simulink model "operationalSpaceInverseDynamicsControl_admittance_compact"  (R2021a)
settings: Solver=VariableStepAuto  StartTime=0.0  StopTime=25  RelTol=1e-3
values from neighbouring files (symbols this model uses):
  K = diag([0 10 0 0 0 10])    [assignment13_main.m]
  Kd = 20*diag([10, 10, 10, 10, 10, 10])    [assignment13_main.m]
  Kd_t = 1*diag([10, 10, 10, 10, 10, 10])    [assignment13_main.m]
  Kp = 50*diag([10, 10, 10, 10, 10, 10])    [assignment13_main.m]
  Kp_t = 5*diag([10, 10, 10, 10, 10, 10])    [assignment13_main.m]
  M_d = 0.1*diag([10 10 10 10 10 10])    [assignment13_main.m]
  M_t = 0.05*diag([10 10 10 10 10 10])    [assignment13_main.m]
  x_d_const = [numeric_dk(1:3,4) ... (first row only)    [assignment13_main.m]
libraries: vrlib x1, robotcorelib x1
settings Model: Creator=fabio  LastModifiedBy=fabio

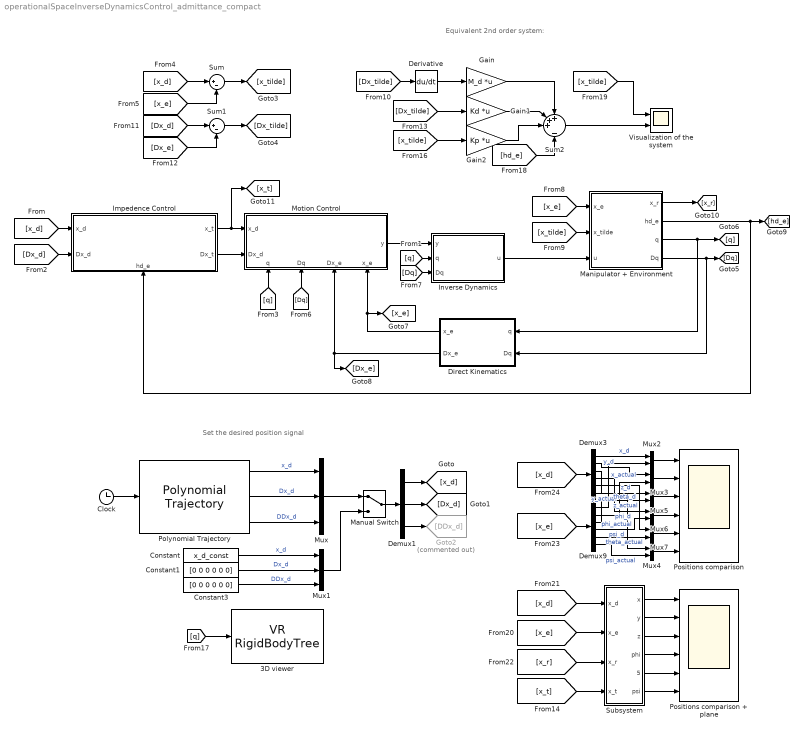
== system operationalSpaceInverseDynamicsControl_admittance_compact ==
  note: Set the desired position signal
  note: Equivalent 2nd order system:
  3D viewer : vrlib/VR RigidBodyTree  RBT=robot  useRBT=off  Ts=0.5  ForceViewerOpen=on
      settings: SourceProductBaseCode=SL
  Clock : Clock
  Constant : Constant  Value=x_d_const
  Constant1 : Constant  Value=[0 0 0 0 0 0]
  Constant3 : Constant  Value=[0 0 0 0 0 0]
  Demux1 : Demux  Outputs=3
  Demux3 : Demux  Outputs=6
  Demux9 : Demux  Outputs=6
  Derivative : Derivative
  Direct Kinematics : Subsystem
  Gain : Gain  Gain=M_d  Multiplication=Matrix(K*u)
  Gain1 : Gain  Gain=Kd  Multiplication=Matrix(K*u)
  Gain2 : Gain  Gain=Kp  Multiplication=Matrix(K*u)
  Goto2 : Goto  Commented=on  GotoTag=DDx_d
  Impedence Control : Subsystem
      settings: PortSchema="{\"entries\":[{\"content\":{\"sides\":[{\"content\":{\"connectorIds\":[\"In1\",\"In2\"]},\"type\":\"ConnectorPlacement.EquallySpacedRectSide\",\"uuid\":\"4a21bbab-43a7-495a-80bb-06e5f1d5644f\"},{\"content\":{\"connectorIds\":[\"Out1\",\"Out2\"],\"side\":\"RIGHT\"},\"type\":\"ConnectorPlacement.EquallySpacedRectSide\",\"uuid\":\"408d256b-dc21-48d5-8048-0ab1741a41e2\"},{\"content\":{\"connectorIds\":[],\"side\":\"TOP\"},\"type\":\"ConnectorPlacement.EquallySpacedRectSide\",\"uuid\":\"05326777-d73e-456a-8a24-eec595721ebb\"},{\"content\":{\"connectorIds\":[\"In3\"],\"side\":\"BOTTOM\"},\"type\":\"ConnectorPlacement.EquallySpacedRectSide\",\"uuid\":\"d6ac4636-ecb5-40e1-909e-b7ba41c5dbf6\"}]},\"type\":\"ConnectorPlacement.EquallySpacedConnector\",\"uuid\":\"f5a6fa07-c06e-4cca-970a-a576f537631e\"}],\"packageUris\":[\"http://schema.mathworks.com/mf0/Connector/R2020b\"],\"version\":\"1.0\"}"
  Inverse Dynamics : Subsystem
  Manipulator + Environment : Subsystem
  Manual Switch : ManualSwitch
  Motion Control : Subsystem
      settings: PortSchema="{\"entries\":[{\"content\":{\"sides\":[{\"content\":{\"connectorIds\":[\"In1\",\"In2\"]},\"type\":\"ConnectorPlacement.EquallySpacedRectSide\",\"uuid\":\"4a21bbab-43a7-495a-80bb-06e5f1d5644f\"},{\"content\":{\"connectorIds\":[\"Out1\"],\"side\":\"RIGHT\"},\"type\":\"ConnectorPlacement.EquallySpacedRectSide\",\"uuid\":\"408d256b-dc21-48d5-8048-0ab1741a41e2\"},{\"content\":{\"connectorIds\":[],\"side\":\"TOP\"},\"type\":\"ConnectorPlacement.EquallySpacedRectSide\",\"uuid\":\"05326777-d73e-456a-8a24-eec595721ebb\"},{\"content\":{\"connectorIds\":[\"In3\",\"In4\",\"In5\",\"In6\"],\"side\":\"BOTTOM\"},\"type\":\"ConnectorPlacement.EquallySpacedRectSide\",\"uuid\":\"d6ac4636-ecb5-40e1-909e-b7ba41c5dbf6\"}]},\"type\":\"ConnectorPlacement.EquallySpacedConnector\",\"uuid\":\"f5a6fa07-c06e-4cca-970a-a576f537631e\"}],\"packageUris\":[\"http://schema.mathworks.com/mf0/Connector/R2020b\"],\"version\":\"1.0\"}"
  Mux : Mux  Inputs=3
  Mux1 : Mux  Inputs=3
  Mux{2..7} (6 alike) : Mux  Inputs=2
  Polynomial Trajectory : robotcorelib/Polynomial Trajectory  WaypointSource=Internal  Waypoints=x_d  TimePoints=[ 0, 10, 20]  TimeInterval=[ 1, 4 ]  Method=Cubic Polynomial  ParameterSource=Internal  VelocityBoundaryCondition=zeros( 6, 3)  AccelerationBoundaryCondition=zeros( 2, 5 )  SimulateUsing=Interpreted execution
  Positions comparison : Scope  NumInputPorts=6
  Positions comparison + plane : Scope  NumInputPorts=6
  Subsystem : Subsystem
  Sum : Sum  Inputs=|+-
  Sum1 : Sum  Inputs=|+-
  Sum2 : Sum  Inputs=+++|-
  Visualization of the system : Scope  NumInputPorts=2
  wires:
  Clock/1 -> Polynomial Trajectory/1
  Polynomial Trajectory/2 -> Mux/2  "Dx_d"
  Polynomial Trajectory/1 -> Mux/1  "x_d"
  Polynomial Trajectory/3 -> Mux/3  "DDx_d"
  Mux/1 -> Manual Switch/1
  Manual Switch/1 -> Demux1/1
  Demux1/1 -> [x_d]
  Demux1/2 -> [Dx_d]
  Demux1/3 -> Goto2/1
  Constant/1 -> Mux1/1  "x_d"
  Constant1/1 -> Mux1/2  "Dx_d"
  Mux1/1 -> Manual Switch/2
  Constant3/1 -> Mux1/3  "DDx_d"
  [q] -> 3D viewer/1
  Manipulator + Environment/4(Dq) -> Direct Kinematics/2(Dq), [Dq]
  Manipulator + Environment/3(q) -> Direct Kinematics/1(q), [q]
  Inverse Dynamics/1(u) -> Manipulator + Environment/3(u)
  [q] -> Inverse Dynamics/2(q)
  [Dq] -> Inverse Dynamics/3(Dq)
  Manipulator + Environment/2(hd_e) -> Impedence Control/3(hd_e), [hd_e]
  Direct Kinematics/2(Dx_e) -> [Dx_e], Motion Control/5(Dx_e)
  Direct Kinematics/1(x_e) -> [x_e], Motion Control/6(x_e)
  [x_d] -> Sum/1
  [x_e] -> Sum/2
  Sum/1 -> [x_tilde]
  [x_e] -> Manipulator + Environment/1(x_e)
  [x_tilde] -> Manipulator + Environment/2(x_tilde)
  [Dx_tilde] -> Derivative/1
  Sum1/1 -> [Dx_tilde]
  [Dx_d] -> Sum1/1
  [Dx_e] -> Sum1/2
  Derivative/1 -> Gain/1
  Gain/1 -> Sum2/1
  [Dx_tilde] -> Gain1/1
  Gain1/1 -> Sum2/2
  [x_tilde] -> Gain2/1
  Gain2/1 -> Sum2/3
  [hd_e] -> Sum2/4
  [x_tilde] -> Visualization of the system/1
  Sum2/1 -> Visualization of the system/2
  [x_d] -> Impedence Control/1(x_d)
  [Dx_d] -> Impedence Control/2(Dx_d)
  Impedence Control/1(x_t) -> [x_t], Motion Control/1(x_d)
  Impedence Control/2(Dx_t) -> Motion Control/2(Dx_d)
  [q] -> Motion Control/3("q  ")
  [Dq] -> Motion Control/4(Dq)
  Motion Control/1(y) -> Inverse Dynamics/1(y)
  Subsystem/5(theta) -> Positions comparison + plane/5
  Subsystem/4(phi) -> Positions comparison + plane/4
  [x_e] -> Subsystem/2(x_e)
  Subsystem/2(y) -> Positions comparison + plane/2
  [x_r] -> Subsystem/3(x_r)
  Subsystem/1(x) -> Positions comparison + plane/1
  Subsystem/3(z) -> Positions comparison + plane/3
  Subsystem/6(psi) -> Positions comparison + plane/6
  [x_d] -> Subsystem/1(x_d)
  [x_e] -> Demux9/1
  Demux9/3 -> Mux5/2  "z_actual"
  Demux9/1 -> Mux2/2  "x_actual"
  [x_d] -> Demux3/1
  Demux3/2 -> Mux3/1  "y_d"
  Demux9/4 -> Mux6/2  "phi_actual"
  Mux7/1 -> Positions comparison/5
  Mux4/1 -> Positions comparison/6
  Demux9/5 -> Mux7/2  "theta_actual"
  Mux2/1 -> Positions comparison/1
  Demux9/6 -> Mux4/2  "psi_actual"
  Demux3/4 -> Mux6/1  "phi_d"
  Mux5/1 -> Positions comparison/3
  Mux6/1 -> Positions comparison/4
  Demux9/2 -> Mux3/2  "y_actual"
  Demux3/6 -> Mux4/1  "psi_d"
  Demux3/1 -> Mux2/1  "x_d"
  Demux3/3 -> Mux5/1  "z_d"
  Mux3/1 -> Positions comparison/2
  Demux3/5 -> Mux7/1  "theta_d"
  Manipulator + Environment/1(x_r) -> [x_r]
  [x_t] -> Subsystem/4(x_t)

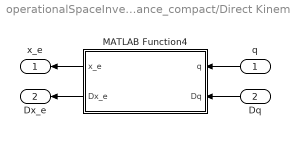
== system operationalSpaceInverseDynamicsControl_admittance_compact/Direct Kinematics ==
  q : Inport
  Dq : Inport  Port=2
  MATLAB Function4 : MATLAB Function  TreatAsAtomicUnit=on
  x_e : Outport
  Dx_e : Outport  Port=2
  wires:
  MATLAB Function4/1(x_e) -> x_e/1
  q/1 -> MATLAB Function4/1(q)
  Dq/1 -> MATLAB Function4/2(Dq)
  MATLAB Function4/2(Dx_e) -> Dx_e/1

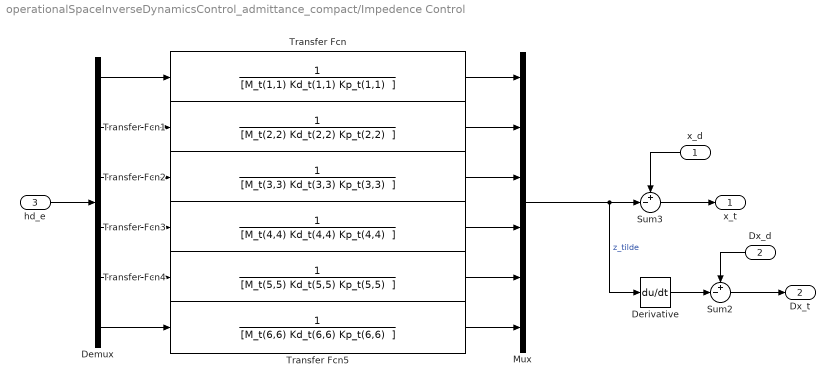
== system operationalSpaceInverseDynamicsControl_admittance_compact/Impedence Control ==
  x_d : Inport
  Dx_d : Inport  Port=2
  hd_e : Inport  Port=3
  Demux : Demux  Outputs=6
  Derivative : Derivative
  Mux : Mux  Inputs=6
  Sum2 : Sum  Inputs=+-|
  Sum3 : Sum  Inputs=+-|
  Transfer Fcn : TransferFcn  Numerator=1  Denominator="[M_t(1,1) Kd_t(1,1) Kp_t(1,1)  ]"
  Transfer Fcn1 : TransferFcn  Numerator=1  Denominator="[M_t(2,2) Kd_t(2,2) Kp_t(2,2)  ]"
  Transfer Fcn2 : TransferFcn  Numerator=1  Denominator="[M_t(3,3) Kd_t(3,3) Kp_t(3,3)  ]"
  Transfer Fcn3 : TransferFcn  Numerator=1  Denominator="[M_t(4,4) Kd_t(4,4) Kp_t(4,4)  ]"
  Transfer Fcn4 : TransferFcn  Numerator=1  Denominator="[M_t(5,5) Kd_t(5,5) Kp_t(5,5)  ]"
  Transfer Fcn5 : TransferFcn  Numerator=1  Denominator="[M_t(6,6) Kd_t(6,6) Kp_t(6,6)  ]"
  x_t : Outport
  Dx_t : Outport  Port=2
  wires:
  x_d/1 -> Sum3/1
  hd_e/1 -> Demux/1
  Demux/1 -> Transfer Fcn/1
  Demux/2 -> Transfer Fcn1/1
  Demux/3 -> Transfer Fcn2/1
  Demux/4 -> Transfer Fcn3/1
  Demux/5 -> Transfer Fcn4/1
  Demux/6 -> Transfer Fcn5/1
  Transfer Fcn/1 -> Mux/1
  Transfer Fcn1/1 -> Mux/2
  Transfer Fcn2/1 -> Mux/3
  Transfer Fcn3/1 -> Mux/4
  Transfer Fcn4/1 -> Mux/5
  Transfer Fcn5/1 -> Mux/6
  Mux/1 -> Derivative/1, Sum3/2  "z_tilde"
  Sum3/1 -> x_t/1
  Sum2/1 -> Dx_t/1
  Dx_d/1 -> Sum2/1
  Derivative/1 -> Sum2/2

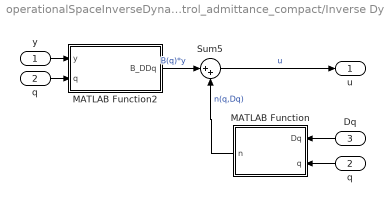
== system operationalSpaceInverseDynamicsControl_admittance_compact/Inverse Dynamics ==
  y : Inport
  q : Inport  Port=2
  Dq : Inport  Port=3
  MATLAB Function : MATLAB Function  TreatAsAtomicUnit=on
  MATLAB Function2 : MATLAB Function  TreatAsAtomicUnit=on
  Sum5 : Sum  Inputs=|++
  "q " : InportShadow  Port=2
  u : Outport
  wires:
  q/1 -> MATLAB Function/2(q)
  MATLAB Function/1(n) -> Sum5/2  "n(q,Dq)"
  "q "/1 -> MATLAB Function2/2(q)
  Dq/1 -> MATLAB Function/1(Dq)
  MATLAB Function2/1(B_DDq) -> Sum5/1  "B(q)*y"
  Sum5/1 -> u/1  "u"
  y/1 -> MATLAB Function2/1(y)

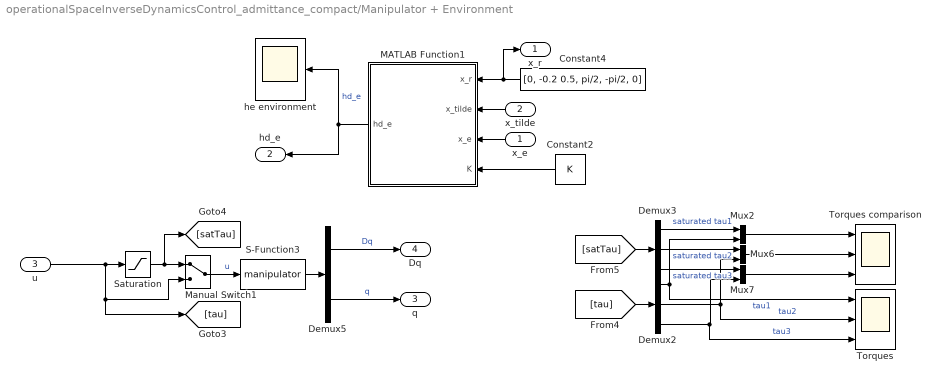
== system operationalSpaceInverseDynamicsControl_admittance_compact/Manipulator + Environment ==
  x_e : Inport
  x_tilde : Inport  Port=2
  u : Inport  Port=3
  Constant2 : Constant  Value=K  VectorParams1D=off
  Constant4 : Constant  Value=[0, -0.2 0.5, pi/2, -pi/2, 0]
  Demux2 : Demux  Outputs=3
  Demux3 : Demux  Outputs=3
  Demux5 : Demux  Outputs=[3 3]
  MATLAB Function1 : MATLAB Function  TreatAsAtomicUnit=on
  Manual Switch1 : ManualSwitch
  Mux2 : Mux  Inputs=2
  Mux6 : Mux  Inputs=2
  Mux7 : Mux  Inputs=2
  S-Function3 : S-Function  FunctionName=manipulator  Parameters=myRobot  SFunctionDeploymentMode=off  EnableBusSupport=off
  Saturation : Saturate  UpperLimit=20  LowerLimit=-20
  Torques : Scope  NumInputPorts=3
  Torques comparison : Scope  NumInputPorts=3
  he environment : Scope
  x_r : Outport
  hd_e : Outport  Port=2
  q : Outport  Port=3
  Dq : Outport  Port=4
  wires:
  u/1 -> Manual Switch1/2, [tau], Saturation/1
  S-Function3/1 -> Demux5/1
  Manual Switch1/1 -> S-Function3/1  "u"
  Saturation/1 -> [satTau], Manual Switch1/1
  x_e/1 -> MATLAB Function1/3(x_e)
  Demux5/2 -> q/1  "q"
  MATLAB Function1/1(hd_e) -> hd_e/1, he environment/1  "hd_e"
  Demux5/1 -> Dq/1  "Dq"
  Constant2/1 -> MATLAB Function1/4(K)
  x_tilde/1 -> MATLAB Function1/2(x_tilde)
  Constant4/1 -> x_r/1, MATLAB Function1/1(x_r)
  Demux2/3 -> Torques/3, Mux7/2  "tau3"
  Demux3/2 -> Mux6/1  "saturated tau2"
  Demux3/3 -> Mux7/1  "saturated tau3"
  Demux3/1 -> Mux2/1  "saturated tau1"
  Mux2/1 -> Torques comparison/1
  [satTau] -> Demux3/1
  Mux7/1 -> Torques comparison/3
  Demux2/1 -> Torques/1, Mux2/2  "tau1"
  [tau] -> Demux2/1
  Mux6/1 -> Torques comparison/2
  Demux2/2 -> Torques/2, Mux6/2  "tau2"

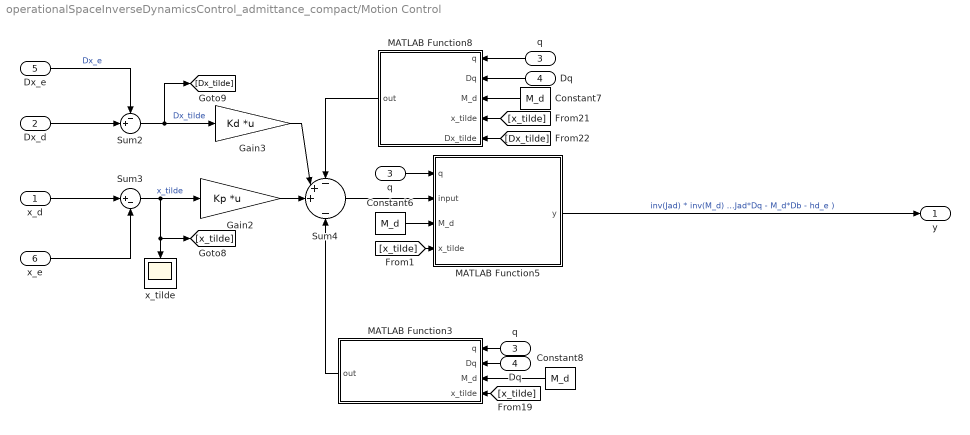
== system operationalSpaceInverseDynamicsControl_admittance_compact/Motion Control ==
  x_d : Inport
  Dx_d : Inport  Port=2
  "q  " : Inport  Port=3
  Dq : Inport  Port=4
  Dx_e : Inport  Port=5
  x_e : Inport  Port=6
  Constant6 : Constant  Value=M_d  VectorParams1D=off
  Constant7 : Constant  Value=M_d  VectorParams1D=off
  Constant8 : Constant  Value=M_d  VectorParams1D=off
  "Dq " : InportShadow  Port=4
  Gain2 : Gain  Gain=Kp  Multiplication=Matrix(K*u) (u vector)
  Gain3 : Gain  Gain=Kd  Multiplication=Matrix(K*u) (u vector)
  MATLAB Function3 : MATLAB Function  TreatAsAtomicUnit=on
  MATLAB Function5 : MATLAB Function  TreatAsAtomicUnit=on
  MATLAB Function8 : MATLAB Function  TreatAsAtomicUnit=on
  Sum2 : Sum  Inputs=-+|
  Sum3 : Sum  Inputs=|+-
  Sum4 : Sum  Inputs=-++|-
  "q " : InportShadow  Port=3
  "q   " : InportShadow  Port=3
  x_tilde : Scope
  y : Outport
  wires:
  [x_tilde] -> MATLAB Function3/4(x_tilde)
  MATLAB Function3/1(out) -> Sum4/4
  Sum3/1 -> Gain2/1, [x_tilde], x_tilde/1  "x_tilde"
  x_e/1 -> Sum3/2
  Constant6/1 -> MATLAB Function5/3(M_d)
  "q   "/1 -> MATLAB Function5/1(q)
  "q "/1 -> MATLAB Function3/1(q)
  Gain3/1 -> Sum4/2
  Dq/1 -> MATLAB Function3/2(Dq)
  Dx_e/1 -> Sum2/1  "Dx_e"
  Constant8/1 -> MATLAB Function3/3(M_d)
  Sum4/1 -> MATLAB Function5/2(input)
  Sum2/1 -> [Dx_tilde], Gain3/1  "Dx_tilde"
  Gain2/1 -> Sum4/3
  x_d/1 -> Sum3/1
  Dx_d/1 -> Sum2/2
  MATLAB Function5/1(y) -> y/1  "inv(Jad) * inv(M_d) * ( Kd*Dx_tilde + Kp*x_tilde - M_d*DJad*Dq - M_d*Db - hd_e )"
  [x_tilde] -> MATLAB Function8/4(x_tilde)
  "q  "/1 -> MATLAB Function8/1(q)
  "Dq "/1 -> MATLAB Function8/2(Dq)
  Constant7/1 -> MATLAB Function8/3(M_d)
  [Dx_tilde] -> MATLAB Function8/5(Dx_tilde)
  MATLAB Function8/1(out) -> Sum4/1
  [x_tilde] -> MATLAB Function5/4(x_tilde)

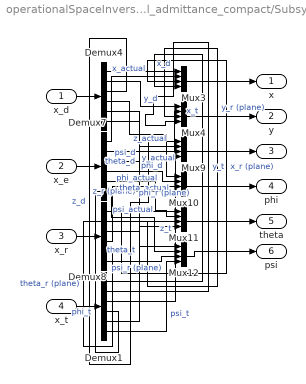
== system operationalSpaceInverseDynamicsControl_admittance_compact/Subsystem ==
  x_d : Inport
  x_e : Inport  Port=2
  x_r : Inport  Port=3
  x_t : Inport  Port=4
  Demux{1,4,7..8} (4 alike) : Demux  Outputs=6
  Mux{3..4,9..12} (6 alike) : Mux
  x : Outport
  y : Outport  Port=2
  z : Outport  Port=3
  phi : Outport  Port=4
  theta : Outport  Port=5
  psi : Outport  Port=6
  wires:
  Demux8/1 -> Mux3/3  "x_r (plane)"
  Demux7/3 -> Mux9/2  "z_actual"
  Demux4/4 -> Mux10/1  "phi_d"
  Demux8/2 -> Mux4/3  "y_r (plane)"
  Demux7/6 -> Mux12/2  "psi_actual"
  Demux7/4 -> Mux10/2  "phi_actual"
  Demux7/1 -> Mux3/2  "x_actual"
  Demux8/3 -> Mux9/3  "z_r (plane)"
  Demux4/3 -> Mux9/1  "z_d"
  Demux4/6 -> Mux12/1  "psi_d"
  Demux4/5 -> Mux11/1  "theta_d"
  Demux7/5 -> Mux11/2  "theta_actual"
  Demux4/2 -> Mux4/1  "y_d"
  Demux4/1 -> Mux3/1  "x_d"
  Demux7/2 -> Mux4/2  "y_actual"
  Demux8/6 -> Mux12/3  "psi_r (plane)"
  Demux8/4 -> Mux10/3  "phi_r (plane)"
  Mux11/1 -> theta/1
  Demux8/5 -> Mux11/3  "theta_r (plane)"
  x_d/1 -> Demux4/1
  x_e/1 -> Demux7/1
  Mux9/1 -> z/1
  Mux12/1 -> psi/1
  Mux10/1 -> phi/1
  Mux4/1 -> y/1
  Mux3/1 -> x/1
  x_r/1 -> Demux8/1
  x_t/1 -> Demux1/1
  Demux1/1 -> Mux3/4  "x_t"
  Demux1/2 -> Mux4/4  "y_t"
  Demux1/3 -> Mux9/4  "z_t"
  Demux1/4 -> Mux10/4  "phi_t"
  Demux1/5 -> Mux11/4  "theta_t"
  Demux1/6 -> Mux12/4  "psi_t"

== matlab function operationalSpaceInverseDynamicsControl_admittance_compact/Manipulator + Environment/MATLAB Function1 ==
  data: x_r input; x_tilde input; x_e input; K input; hd_e output
function hd_e  = environment(x_r, x_tilde, x_e, K)
    
    phi_d_e = -x_tilde(4:6);
    
    %Compute T(phi_d_e) function of the euler angles of x_d
    T = [0, -sin(phi_d_e(1)), cos(phi_d_e(1))*sin(phi_d_e(2));
         0,  cos(phi_d_e(1)), sin(phi_d_e(1))*sin(phi_d_e(2));
         1,     0           , cos(phi_d_e(2))                ];

    Ta = [1 0 0   0 0 0 ;
          0 1 0   0 0 0 ;
          0 0 1   0 0 0 ;
          0 0 0 , T(1,:);
          0 0 0 , T(2,:);
          0 0 0 , T(3,:)];    
   
    
    y_plane = x_r(2);
    %contact with the plane
    if max(size(x_e)) > 1 && x_e(2) < y_plane 
        dx_re = x_e - x_r;
        h_e = K * dx_re;
    else %no contact with the plane
        h_e = [0 0 0 0 0 0].';
    end
    
    hd_e = Ta.'*h_e;
end

== matlab function operationalSpaceInverseDynamicsControl_admittance_compact/Inverse Dynamics/MATLAB Function ==
  data: Dq input; n output; q input
function n = n_q_Dq(Dq, q)
    
    %To get the "perfect" matrices use the following code
    C = get_C_matrix(q,Dq);
    G = get_G_matrix(q);
    
    
    %To get the "wrongly estimated" matrices use the following code   
%     theta2 = q(2);   d3 = q(3); 
%     Dtheta2 = Dq(2); Dd3 = Dq(3); 
%     
%     m_Link4 = 0.16;  %0.2kg is the correct value
% 
%     C = [0,                         0,                        0;
%          0,            m_Link4*Dd3*d3,       m_Link4*Dtheta2*d3;
%          0,       -m_Link4*Dtheta2*d3,                        0];
%    
%     G = [           0                           ;
%          (981*m_Link4*sin(theta2)*d3)/100 ;
%           -(981*m_Link4*cos(theta2))/100    ];


    
    n = C*Dq + G; %F = friction is neglected

end

== matlab function operationalSpaceInverseDynamicsControl_admittance_compact/Inverse Dynamics/MATLAB Function2 ==
  data: y input; B_DDq output; q input
function B_DDq = B_q(y,q)
    B_DDq = get_B_matrix(q)*y;
end

== matlab function operationalSpaceInverseDynamicsControl_admittance_compact/Motion Control/MATLAB Function3 ==
  data: q input; out output; Dq input; M_d input; x_tilde input
function out = Md_x_DJad_x_Dq(q, Dq, M_d, x_tilde)
    
    DJad = get_DJad_matrix(q, Dq, x_tilde);
    
    out = M_d * DJad * Dq;
      
end

== matlab function operationalSpaceInverseDynamicsControl_admittance_compact/Direct Kinematics/MATLAB Function4 ==
  data: q input; x_e output; Dx_e output; Dq input
function [x_e, Dx_e] = k(q, Dq) 
    %Compute the direct kinematics from last transformation matrix
    if max(size(q)) < 3
        q = [0 0 0];   
    end
    if max(size(Dq)) < 3
        Dq = [0 0 0];   
    end
    
    %get rotation matrix and translation vector from ∑0 to ∑ee   
    T0_to_ee = get_T0_ee_matrix(q);
    R0_to_ee = T0_to_ee(1:3,1:3);
    p0_to_ee = T0_to_ee(1:3,4);    
                 
    eulerAngles = rotm2eul(R0_to_ee, 'ZYZ');
  
    x_e = [ p0_to_ee;
          eulerAngles.' ]; %return complete direct kinematics
      
    Ja = get_Ja_matrix(q);
    Dx_e = Ja * Dq;
end

== matlab function operationalSpaceInverseDynamicsControl_admittance_compact/Motion Control/MATLAB Function5 ==
  data: q input; y output; input input; M_d input; x_tilde input
function y = invJad_x_invMd(q, input, M_d, x_tilde)
    if max(size(q)) < 3
        q = [0 0 0];   
    end
   
    Jad = get_Jad_matrix(q, x_tilde);
    
    y = pinv(Jad) * inv(M_d) * input;
 
end

== matlab function operationalSpaceInverseDynamicsControl_admittance_compact/Motion Control/MATLAB Function8 ==
  data: q input; out output; Dq input; M_d input; x_tilde input; Dx_tilde input
function out = Md_x_Db(q, Dq, M_d, x_tilde, Dx_tilde)
    
    Jad = get_Jad_matrix(q, x_tilde);
    
    %According to slide 29: 
    Db = (Dx_tilde + Jad*Dq);
    out = M_d * Db;
      
end
